simulink model "part1"  (R2021a)
settings: Solver=VariableStepAuto  StartTime=-0.02  StopTime=0.02  MaxStep=1e-6  RelTol=1e-3
settings Model: Creator=swarn  LastModifiedBy=mansi
settings SolverCC: AlgebraicLoopSolver=TrustRegion
settings DebuggingCC: AlgebraicLoopMsg=none  SFMachineParentedDataDiag=warning

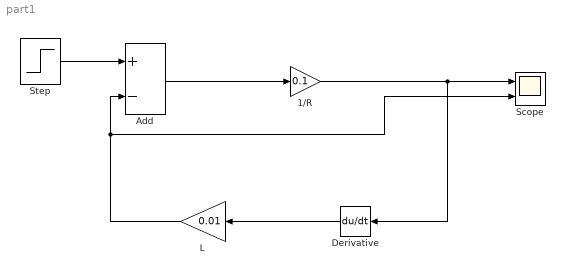
== system part1 ==
  1/R : Gain  Gain=0.1
  Add : Sum  Inputs=+-
  Derivative : Derivative
  L : Gain  Gain=0.01
  Scope : Scope  NumInputPorts=2
  Step : Step  Time=0  SampleTime=0
  wires:
  Step/1 -> Add/1
  Add/1 -> 1/R/1
  1/R/1 -> Derivative/1, Scope/1
  Derivative/1 -> L/1
  L/1 -> Scope/2, Add/2
